simulink model "mavsim"  (R2020a)
settings: Solver=ode45  StartTime=0.0  StopTime=500  RelTol=1e-3  EnableMultiTasking=on
PreLoadFcn:
  | kalman_covariances
InitFcn:
  | param_quad
model workspace (MAT data in the model file):
  traj_x = [0 0.201 0.4 0.601 0.8 1 1.2 1.4 1.6 1.801 2 2.2 ... (4684 elements, 2342x2)]
  traj_y = [0 0.201 0.4 0.601 0.8 1 1.2 1.4 1.6 1.801 2 2.2 ... (4684 elements, 2342x2)]
  traj_z = [0 0.201 0.4 0.601 0.8 1 1.2 1.4 1.6 1.801 2 2.2 ... (4684 elements, 2342x2)]
  vel_x = [0 0 0.201 0.4 0.601 0.8 1 1.2 1.4 1.6 1.801 2 ... (4686 elements, 2343x2)]
  vel_y = [0 0 0.201 0.4 0.601 0.8 1 1.2 1.4 1.6 1.801 2 ... (4686 elements, 2343x2)]
  vel_z = [0 0 0.201 0.4 0.601 0.8 1 1.2 1.4 1.6 1.801 2 ... (4686 elements, 2343x2)]
undefined symbols (not defined in the file or in its folder): airdata, drawAircraft, P, plotmavstatevariables
libraries: simulink x5, sharedTrackingLibrary x1
(part 2 of 2)

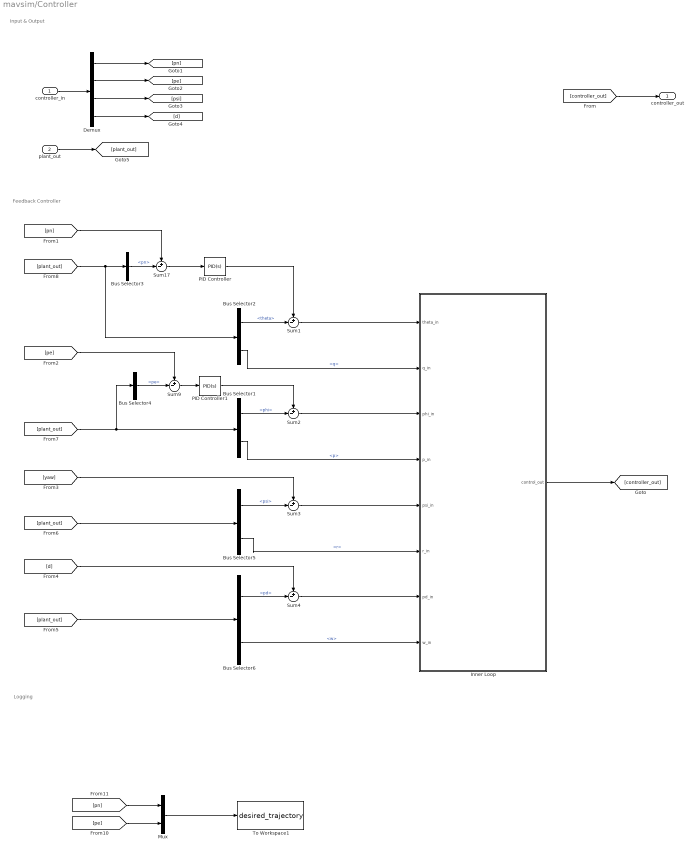
== system mavsim/Controller ==
  note: Logging
  note: Input & Output
  note: Feedback Controller
  controller_in : Inport
  plant_out : Inport  Port=2
  Bus Selector1 : BusSelector  OutputSignals=phi,p
  Bus Selector2 : BusSelector  OutputSignals=theta,q
  Bus Selector3 : BusSelector  OutputSignals=pn
  Bus Selector4 : BusSelector  OutputSignals=pe
  Bus Selector5 : BusSelector  OutputSignals=psi,r
  Bus Selector6 : BusSelector  OutputSignals=pd,w
  Demux : Demux
  Inner Loop : Subsystem
  Mux : Mux  Inputs=2
  PID Controller : simulink/Continuous/PID Controller  Controller=PID  Form=Parallel  TimeDomain=Continuous-time  UseExternalTs=off  SampleTime=1  IntegratorMethod=Forward Euler  FilterMethod=Forward Euler  ControllerParametersSource=internal  P=4.0023736850835e-05  I=2.85008847395968e-08  D=0.0124881440151142  UseFilter=on  N=13.9495577511828  TunerSelectOption=Transfer Function Based (PID Tuner App)  InitialConditionSource=internal  InitialConditionForIntegrator=0  InitialConditionForFilter=0  DifferentiatorICPrevScaledInput=0  ExternalReset=none  TrackingMode=off  Kt=1  LimitOutput=off  UpperSaturationLimit=inf  LowerSaturationLimit=-inf  LinearizeAsGain=on  AntiWindupMode=none  Kb=1  POutMin=[]  POutMax=[]  IOutMin=[]  IOutMax=[]  DOutMin=[]  DOutMax=[]  NOutMin=[]  NOutMax=[]  SumOutMin=[]  SumOutMax=[]  SaturationOutMin=[]  SaturationOutMax=[]  PParamMin=[]  PParamMax=[]  IParamMin=[]  IParamMax=[]  DParamMin=[]  DParamMax=[]  NParamMin=[]  NParamMax=[]  KbParamMin=[]  KbParamMax=[]  KtParamMin=[]  KtParamMax=[]  KbOutMin=[]  KbOutMax=[]  KtOutMin=[]  KtOutMax=[]  IntegratorOutMin=[]  IntegratorOutMax=[]  FilterOutMin=[]  FilterOutMax=[]  SumI1OutMin=[]  SumI1OutMax=[]  SumI2OutMin=[]  SumI2OutMax=[]  SumI3OutMin=[]  SumI3OutMax=[]  SumI4OutMin=[]  SumI4OutMax=[]  SumDOutMin=[]  SumDOutMax=[]  DifferentiatorOutMin=[]  DifferentiatorOutMax=[]  FilterDiffOutCoefMin=[]  FilterDiffOutCoefMax=[]  ReciprocalOutMin=[]  ReciprocalOutMax=[]  SumDenOutMin=[]  SumDenOutMax=[]  SumNumOutMin=[]  SumNumOutMax=[]  DivideOutMin=[]  DivideOutMax=[]  UdiffTsProdOutMin=[]  UdiffTsProdOutMax=[]  NTsProdOutMin=[]  NTsProdOutMax=[]  UintegralTsProdOutMin=[]  UintegralTsProdOutMax=[]  UngainTsProdOutMin=[]  UngainTsProdOutMax=[]  IntegratorContinuousStateAttributes=''  IntegratorStateMustResolveToSignalObject=off  IntegratorRTWStateStorageClass=Auto  FilterContinuousStateAttributes=''  FilterStateMustResolveToSignalObject=off  FilterRTWStateStorageClass=Auto  ParallelPVariant=InternalParameters  IdealPVariant=Disabled  IVariant=InternalParameters  DVariant=InternalParameters  IntegratorVariant=Continuous  SatVariant=Disabled  AWVariant=Passthrough  PCopyVariant=Disabled  TRVariant=Disabled  FdbkBlocksVariant=Forward  IdealPFdbkVariant=Disabled  SatFdbkVariant=Disabled  DerivativeFilterVariant=ContFilter  NVariant=InternalParameters  NCopyVariant=Disabled  FilterICVariant=InternalICsFilter  IntegratorICVariant=InternalICs  ExternalResetVariant=Disabled  TRSumVariant=Passthrough  SumFdbkVariant=Disabled  SumVariant=Sum_PID  TsampFilterVariant=InternalTs  TsampNgainVariant=Passthrough  TsampIntegralVariant=Passthrough
  PID Controller1 : simulink/Continuous/PID Controller  Controller=PID  Form=Parallel  TimeDomain=Continuous-time  UseExternalTs=off  SampleTime=1  IntegratorMethod=Forward Euler  FilterMethod=Forward Euler  ControllerParametersSource=internal  P=-3.61891016622515e-05  I=-2.46103907876315e-08  D=-0.0118238269942865  UseFilter=on  N=13.3217242306574  TunerSelectOption=Transfer Function Based (PID Tuner App)  InitialConditionSource=internal  InitialConditionForIntegrator=0  InitialConditionForFilter=0  DifferentiatorICPrevScaledInput=0  ExternalReset=none  TrackingMode=off  Kt=1  LimitOutput=off  UpperSaturationLimit=inf  LowerSaturationLimit=-inf  LinearizeAsGain=on  AntiWindupMode=none  Kb=1  POutMin=[]  POutMax=[]  IOutMin=[]  IOutMax=[]  DOutMin=[]  DOutMax=[]  NOutMin=[]  NOutMax=[]  SumOutMin=[]  SumOutMax=[]  SaturationOutMin=[]  SaturationOutMax=[]  PParamMin=[]  PParamMax=[]  IParamMin=[]  IParamMax=[]  DParamMin=[]  DParamMax=[]  NParamMin=[]  NParamMax=[]  KbParamMin=[]  KbParamMax=[]  KtParamMin=[]  KtParamMax=[]  KbOutMin=[]  KbOutMax=[]  KtOutMin=[]  KtOutMax=[]  IntegratorOutMin=[]  IntegratorOutMax=[]  FilterOutMin=[]  FilterOutMax=[]  SumI1OutMin=[]  SumI1OutMax=[]  SumI2OutMin=[]  SumI2OutMax=[]  SumI3OutMin=[]  SumI3OutMax=[]  SumI4OutMin=[]  SumI4OutMax=[]  SumDOutMin=[]  SumDOutMax=[]  DifferentiatorOutMin=[]  DifferentiatorOutMax=[]  FilterDiffOutCoefMin=[]  FilterDiffOutCoefMax=[]  ReciprocalOutMin=[]  ReciprocalOutMax=[]  SumDenOutMin=[]  SumDenOutMax=[]  SumNumOutMin=[]  SumNumOutMax=[]  DivideOutMin=[]  DivideOutMax=[]  UdiffTsProdOutMin=[]  UdiffTsProdOutMax=[]  NTsProdOutMin=[]  NTsProdOutMax=[]  UintegralTsProdOutMin=[]  UintegralTsProdOutMax=[]  UngainTsProdOutMin=[]  UngainTsProdOutMax=[]  IntegratorContinuousStateAttributes=''  IntegratorStateMustResolveToSignalObject=off  IntegratorRTWStateStorageClass=Auto  FilterContinuousStateAttributes=''  FilterStateMustResolveToSignalObject=off  FilterRTWStateStorageClass=Auto  ParallelPVariant=InternalParameters  IdealPVariant=Disabled  IVariant=InternalParameters  DVariant=InternalParameters  IntegratorVariant=Continuous  SatVariant=Disabled  AWVariant=Passthrough  PCopyVariant=Disabled  TRVariant=Disabled  FdbkBlocksVariant=Forward  IdealPFdbkVariant=Disabled  SatFdbkVariant=Disabled  DerivativeFilterVariant=ContFilter  NVariant=InternalParameters  NCopyVariant=Disabled  FilterICVariant=InternalICsFilter  IntegratorICVariant=InternalICs  ExternalResetVariant=Disabled  TRSumVariant=Passthrough  SumFdbkVariant=Disabled  SumVariant=Sum_PID  TsampFilterVariant=InternalTs  TsampNgainVariant=Passthrough  TsampIntegralVariant=Passthrough
  Sum{1..4,9,17} (6 alike) : Sum  Inputs=+-|
  To Workspace1 : ToWorkspace  VariableName=desired_trajectory  SaveFormat=Timeseries  SampleTime=-1
  controller_out : Outport  VectorParamsAs1DForOutWhenUnconnected=off
  wires:
  [yaw] -> Sum3/1
  [d] -> Sum4/1
  Bus Selector2/1 -> Sum1/2  "<theta>"
  Bus Selector4/1 -> Sum9/2  "<pe>"
  Sum2/1 -> Inner Loop/3(phi_in)
  Sum4/1 -> Inner Loop/7(pd_in)
  PID Controller/1 -> Sum1/1
  Bus Selector2/2 -> Inner Loop/2(q_in)  "<q>"
  Sum17/1 -> PID Controller/1
  Bus Selector5/1 -> Sum3/2  "<psi>"
  Bus Selector6/2 -> Inner Loop/8(w_in)  "<w>"
  Inner Loop/1(control_out) -> [controller_out]
  Bus Selector1/2 -> Inner Loop/4(p_in)  "<p>"
  [pn] -> Sum17/1
  PID Controller1/1 -> Sum2/1
  Sum9/1 -> PID Controller1/1
  Bus Selector1/1 -> Sum2/2  "<phi>"
  Sum1/1 -> Inner Loop/1(theta_in)
  [plant_out] -> Bus Selector6/1
  [pe] -> Sum9/1
  Sum3/1 -> Inner Loop/5(psi_in)
  Bus Selector6/1 -> Sum4/2  "<pd>"
  Bus Selector5/2 -> Inner Loop/6(r_in)  "<r>"
  Bus Selector3/1 -> Sum17/2  "<pn>"
  [controller_out] -> controller_out/1
  Demux/1 -> [pn]
  Demux/2 -> [pe]
  Demux/3 -> [psi]
  Demux/4 -> [d]
  plant_out/1 -> [plant_out]
  [plant_out] -> Bus Selector5/1
  [plant_out] -> Bus Selector4/1, Bus Selector1/1
  [plant_out] -> Bus Selector2/1, Bus Selector3/1
  controller_in/1 -> Demux/1
  [pe] -> Mux/2
  [pn] -> Mux/1
  Mux/1 -> To Workspace1/1

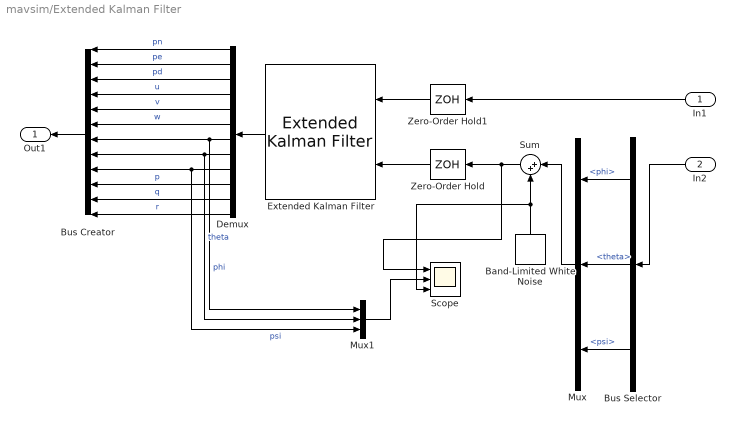
== system mavsim/Extended Kalman Filter ==
  In1 : Inport
  In2 : Inport  Port=2
  Band-Limited White Noise : simulink/Sources/Band-Limited White Noise  Cov=[0.000001 0.000001 0.000001]  Ts=0.005  seed=[23341]
  Bus Creator : BusCreator  Inputs=12
  Bus Selector : BusSelector  OutputSignals=phi,theta,psi
  Demux : Demux  Outputs=12
  Extended Kalman Filter : sharedTrackingLibrary/Extended Kalman Filter  StateTransitionFcn=mavStateTransitionFcn  HasStateTransitionJacobianFcn=off  HasAdditiveProcessNoise=Additive  ProcessNoise=Q  HasTimeVaryingProcessNoise=off  HasStateTransitionFcnExtraArgument=1  InitialState=[0 0 0 0 0 0 0 0 0 0 0 0]  InitialStateCovariance=1e-6  MeasurementFcn1=gyroFcn  HasMeasurementJacobianFcn1=off  HasMeasurementEnablePort1=off  HasAdditiveMeasurementNoise1=Additive  MeasurementNoise1=R  HasTimeVaryingMeasurementNoise1=off  HasMeasurementFcnExtraArgument1=0  MeasurementFcn2=myMeasurementFcn  HasMeasurementJacobianFcn2=off  HasMeasurementEnablePort2=off  HasAdditiveMeasurementNoise2=Additive  MeasurementNoise2=1  HasTimeVaryingMeasurementNoise2=off  HasMeasurementFcnExtraArgument2=0  MeasurementFcn3=myMeasurementFcn  HasMeasurementJacobianFcn3=off  HasMeasurementEnablePort3=off  HasAdditiveMeasurementNoise3=Additive  MeasurementNoise3=1  HasTimeVaryingMeasurementNoise3=off  HasMeasurementFcnExtraArgument3=0  MeasurementFcn4=myMeasurementFcn  HasMeasurementJacobianFcn4=off  HasMeasurementEnablePort4=off  HasAdditiveMeasurementNoise4=Additive  MeasurementNoise4=1  HasTimeVaryingMeasurementNoise4=off  HasMeasurementFcnExtraArgument4=0  MeasurementFcn5=myMeasurementFcn  HasMeasurementJacobianFcn5=off  HasMeasurementEnablePort5=off  HasAdditiveMeasurementNoise5=Additive  MeasurementNoise5=1  HasTimeVaryingMeasurementNoise5=off  HasMeasurementFcnExtraArgument5=0  EnableMultirate=off  StateTransitionFcnSampleTime=1  MeasurementFcn1SampleTime=1  MeasurementFcn2SampleTime=1  MeasurementFcn3SampleTime=1  MeasurementFcn4SampleTime=1  MeasurementFcn5SampleTime=1  UseCurrentEstimator=on  OutputStateCovariance=off  DataType=double  SampleTime=.005  NumberOfMeasurements=1
      settings: SourceProductBaseCode=CT,DR,TF,ID,NV,AR,RO,VE
  Mux : Mux  Inputs=3
  Mux1 : Mux  Inputs=3
  Scope : Scope  NumInputPorts=3
  Sum : Sum  Inputs=|++
  Zero-Order Hold : ZeroOrderHold  SampleTime=.005
  Zero-Order Hold1 : ZeroOrderHold  SampleTime=.005
  Out1 : Outport  VectorParamsAs1DForOutWhenUnconnected=off
  wires:
  Sum/1 -> Scope/1, Zero-Order Hold/1
  Zero-Order Hold/1 -> Extended Kalman Filter/2
  In2/1 -> Bus Selector/1
  Mux/1 -> Sum/1
  In1/1 -> Zero-Order Hold1/1
  Zero-Order Hold1/1 -> Extended Kalman Filter/1
  Extended Kalman Filter/1 -> Demux/1
  Bus Creator/1 -> Out1/1
  Demux/1 -> Bus Creator/1  "pn"
  Demux/2 -> Bus Creator/2  "pe"
  Demux/3 -> Bus Creator/3  "pd"
  Demux/4 -> Bus Creator/4  "u"
  Demux/5 -> Bus Creator/5  "v"
  Demux/6 -> Bus Creator/6  "w"
  Demux/8 -> Mux1/2, Bus Creator/8  "theta"
  Demux/7 -> Mux1/1, Bus Creator/7  "phi"
  Demux/9 -> Mux1/3, Bus Creator/9  "psi"
  Demux/10 -> Bus Creator/10  "p"
  Demux/11 -> Bus Creator/11  "q"
  Demux/12 -> Bus Creator/12  "r"
  Bus Selector/3 -> Mux/3  "<psi>"
  Bus Selector/1 -> Mux/1  "<phi>"
  Bus Selector/2 -> Mux/2  "<theta>"
  Mux1/1 -> Scope/2
  Band-Limited White Noise/1 -> Scope/3, Sum/2

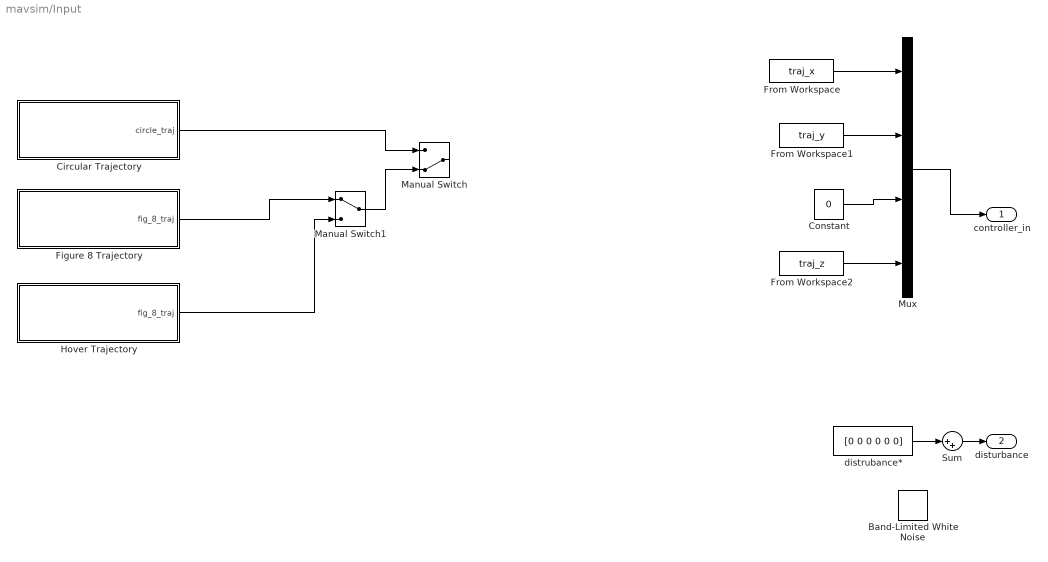
== system mavsim/Input ==
  Band-Limited White Noise : simulink/Sources/Band-Limited White Noise  Cov=[0 0 0 0.0000001 0.0000001 0.0000001]  Ts=0.1  seed=[23341]
  Circular Trajectory : Subsystem
  Constant : Constant  Value=0
  Figure 8 Trajectory : Subsystem
  From Workspace : FromWorkspace  VariableName=traj_x  SampleTime=-1  OutputAfterFinalValue=Holding final value
  From Workspace1 : FromWorkspace  VariableName=traj_y  SampleTime=-1  OutputAfterFinalValue=Holding final value
  From Workspace2 : FromWorkspace  VariableName=traj_z  SampleTime=-1  OutputAfterFinalValue=Holding final value
  Hover Trajectory : Subsystem
  Manual Switch : ManualSwitch  CurrentSetting=0
  Manual Switch1 : ManualSwitch
  Mux : Mux
  Sum : Sum  Inputs=|++
  distrubance* : Constant  Value=[0 0 0 0 0 0]  SampleTime=0
  controller_in : Outport  VectorParamsAs1DForOutWhenUnconnected=off
  disturbance : Outport  Port=2  VectorParamsAs1DForOutWhenUnconnected=off
  wires:
  Circular Trajectory/1(circle_traj) -> Manual Switch/1
  Mux/1 -> controller_in/1
  Sum/1 -> disturbance/1
  distrubance*/1 -> Sum/1
  Figure 8 Trajectory/1(fig_8_traj) -> Manual Switch1/1
  Hover Trajectory/1(fig_8_traj) -> Manual Switch1/2
  Manual Switch1/1 -> Manual Switch/2
  From Workspace2/1 -> Mux/4
  Constant/1 -> Mux/3
  From Workspace1/1 -> Mux/2
  From Workspace/1 -> Mux/1

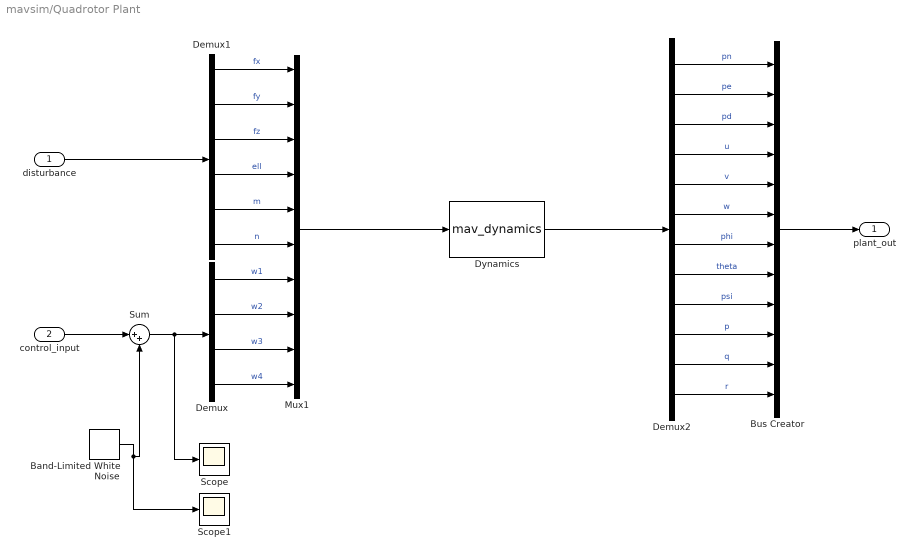
== system mavsim/Quadrotor Plant ==
  disturbance : Inport
  control_input : Inport  Port=2
  Band-Limited White Noise : simulink/Sources/Band-Limited White Noise  Cov=[0.000000009]  Ts=0.005  seed=[23341 4 973 66668]
  Bus Creator : BusCreator  Inputs=12
  Demux : Demux
  Demux1 : Demux  Outputs=6
  Demux2 : Demux  Outputs=12
  Dynamics : S-Function  FunctionName=mav_dynamics  Parameters=P  SFunctionDeploymentMode=off  EnableBusSupport=off
  Mux1 : Mux  Inputs=10
  Scope : Scope
  Scope1 : Scope
  Sum : Sum  Inputs=|++
  plant_out : Outport  VectorParamsAs1DForOutWhenUnconnected=off
  wires:
  Dynamics/1 -> Demux2/1
  Demux2/12 -> Bus Creator/12  "r"
  Demux2/1 -> Bus Creator/1  "pn"
  Demux2/2 -> Bus Creator/2  "pe"
  Demux2/3 -> Bus Creator/3  "pd"
  Demux2/4 -> Bus Creator/4  "u"
  Demux2/5 -> Bus Creator/5  "v"
  Demux2/6 -> Bus Creator/6  "w"
  Demux2/8 -> Bus Creator/8  "theta"
  Demux2/7 -> Bus Creator/7  "phi"
  Demux2/9 -> Bus Creator/9  "psi"
  Demux2/10 -> Bus Creator/10  "p"
  Demux2/11 -> Bus Creator/11  "q"
  Bus Creator/1 -> plant_out/1
  Mux1/1 -> Dynamics/1
  Demux/2 -> Mux1/8  "w2"
  Demux1/5 -> Mux1/5  "m"
  Demux1/4 -> Mux1/4  "ell"
  Demux/4 -> Mux1/10  "w4"
  Demux/1 -> Mux1/7  "w1"
  Demux1/6 -> Mux1/6  "n"
  Demux1/2 -> Mux1/2  "fy"
  Demux1/3 -> Mux1/3  "fz"
  Demux/3 -> Mux1/9  "w3"
  Demux1/1 -> Mux1/1  "fx"
  disturbance/1 -> Demux1/1
  Band-Limited White Noise/1 -> Sum/2, Scope1/1
  control_input/1 -> Sum/1
  Sum/1 -> Scope/1, Demux/1

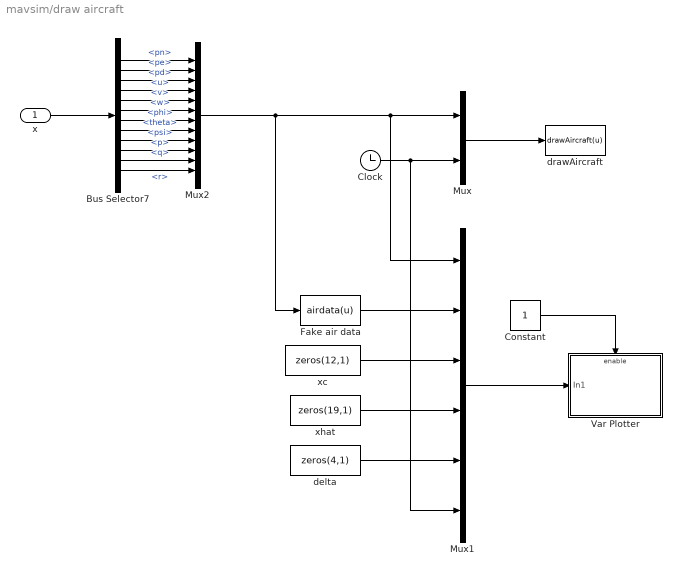
== system mavsim/draw aircraft ==
  x : Inport
  Bus Selector7 : BusSelector  OutputSignals=pn,pe,pd,u,v,w,phi,theta,psi,p,q,r
  Clock : Clock
  Constant : Constant
  Fake air data : MATLABFcn  MATLABFcn=airdata(u)  OutputDimensions=6  SampleTime=0.1
  Mux : Mux  Inputs=2
  Mux1 : Mux  Inputs=6
  Mux2 : Mux  Inputs=12
  Var Plotter : Subsystem
  delta : Constant  Value=zeros(4,1)
  drawAircraft : MATLABFcn  MATLABFcn=drawAircraft(u)  OutputDimensions=0  SampleTime=0.1
  xc : Constant  Value=zeros(12,1)
  xhat : Constant  Value=zeros(19,1)
  wires:
  Mux/1 -> drawAircraft/1
  Mux2/1 -> Fake air data/1, Mux1/1, Mux/1
  Clock/1 -> Mux/2, Mux1/6
  xhat/1 -> Mux1/4
  xc/1 -> Mux1/3
  delta/1 -> Mux1/5
  Fake air data/1 -> Mux1/2
  Mux1/1 -> Var Plotter/1(In1)
  Constant/1 -> Var Plotter/Enable
  Bus Selector7/12 -> Mux2/12  "<r>"
  Bus Selector7/4 -> Mux2/4  "<u>"
  Bus Selector7/9 -> Mux2/9  "<psi>"
  Bus Selector7/5 -> Mux2/5  "<v>"
  Bus Selector7/10 -> Mux2/10  "<p>"
  Bus Selector7/7 -> Mux2/7  "<phi>"
  Bus Selector7/3 -> Mux2/3  "<pd>"
  Bus Selector7/8 -> Mux2/8  "<theta>"
  Bus Selector7/2 -> Mux2/2  "<pe>"
  Bus Selector7/11 -> Mux2/11  "<q>"
  x/1 -> Bus Selector7/1
  Bus Selector7/1 -> Mux2/1  "<pn>"
  Bus Selector7/6 -> Mux2/6  "<w>"

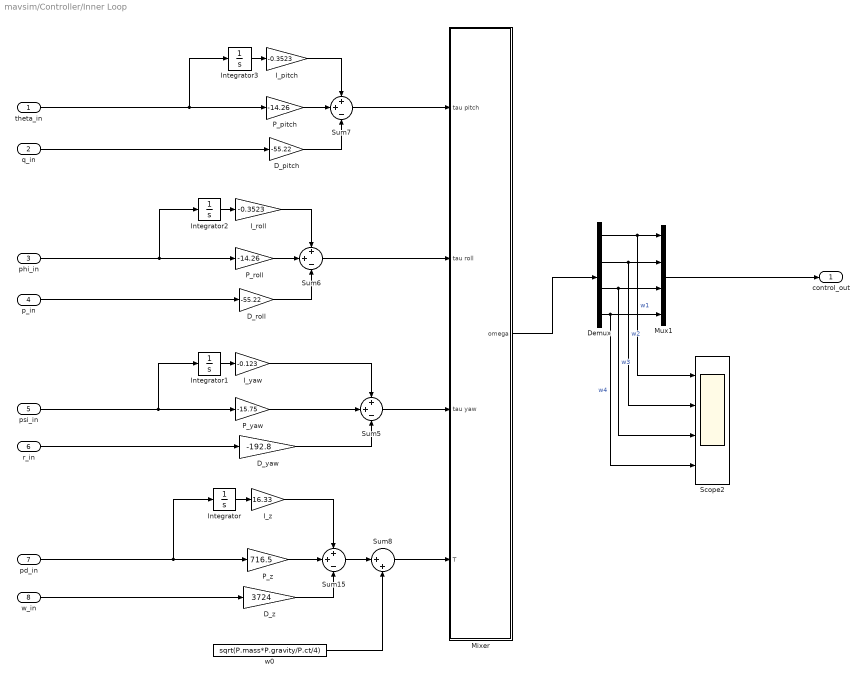
== system mavsim/Controller/Inner Loop ==
  theta_in : Inport
  q_in : Inport  Port=2
  phi_in : Inport  Port=3
  p_in : Inport  Port=4
  psi_in : Inport  Port=5
  r_in : Inport  Port=6
  pd_in : Inport  Port=7
  w_in : Inport  Port=8
  D_pitch : Gain  Gain=-55.22
  D_roll : Gain  Gain=-55.22
  D_yaw : Gain  Gain=-192.8
  D_z : Gain  Gain=3724
  Demux : Demux
  I_pitch : Gain  Gain=-0.3523
  I_roll : Gain  Gain=-0.3523
  I_yaw : Gain  Gain=-0.123
  I_z : Gain  Gain=16.33
  Integrator{,1..3} (4 alike) : Integrator
  Mixer : Subsystem
  Mux1 : Mux
  P_pitch : Gain  Gain=-14.26
  P_roll : Gain  Gain=-14.26
  P_yaw : Gain  Gain=-15.75
  P_z : Gain  Gain=716.5
  Scope2 : Scope  NumInputPorts=4
  Sum{5..7,15} (4 alike) : Sum  Inputs=++-
  Sum8 : Sum  Inputs=|++
  w0 : Constant  Value=sqrt(P.mass*P.gravity/P.ct/4)  SampleTime=0
  control_out : Outport  VectorParamsAs1DForOutWhenUnconnected=off
  wires:
  r_in/1 -> D_yaw/1
  P_pitch/1 -> Sum7/2
  D_yaw/1 -> Sum5/3
  P_roll/1 -> Sum6/2
  Demux/4 -> Mux1/4, Scope2/4  "w4"
  Demux/1 -> Mux1/1, Scope2/1  "w1"
  I_yaw/1 -> Sum5/1
  pd_in/1 -> Integrator/1, P_z/1
  theta_in/1 -> Integrator3/1, P_pitch/1
  Demux/2 -> Mux1/2, Scope2/2  "w2"
  Sum15/1 -> Sum8/1
  I_z/1 -> Sum15/1
  psi_in/1 -> Integrator1/1, P_yaw/1
  Sum8/1 -> Mixer/4(T)
  Mixer/1(omega) -> Demux/1
  phi_in/1 -> Integrator2/1, P_roll/1
  D_roll/1 -> Sum6/3
  Sum7/1 -> Mixer/1(tau pitch)
  Sum5/1 -> Mixer/3(tau yaw)
  Integrator2/1 -> I_roll/1
  Integrator/1 -> I_z/1
  P_yaw/1 -> Sum5/2
  p_in/1 -> D_roll/1
  P_z/1 -> Sum15/2
  Integrator1/1 -> I_yaw/1
  Integrator3/1 -> I_pitch/1
  D_z/1 -> Sum15/3
  D_pitch/1 -> Sum7/3
  Demux/3 -> Mux1/3, Scope2/3  "w3"
  I_pitch/1 -> Sum7/1
  q_in/1 -> D_pitch/1
  w0/1 -> Sum8/2
  I_roll/1 -> Sum6/1
  Mux1/1 -> control_out/1
  Sum6/1 -> Mixer/2(tau roll)
  w_in/1 -> D_z/1

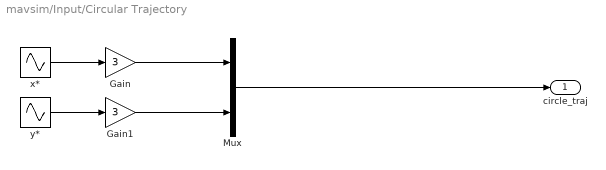
== system mavsim/Input/Circular Trajectory ==
  Gain : Gain  Gain=3
  Gain1 : Gain  Gain=3
  Mux : Mux  Inputs=2
  x* : Sin  Amplitude=50  Frequency=2*pi*.0125  Phase=-pi/2  SampleTime=0
  y* : Sin  Amplitude=50  Frequency=2*pi*.0125  SampleTime=0
  circle_traj : Outport  VectorParamsAs1DForOutWhenUnconnected=off
  wires:
  Mux/1 -> circle_traj/1
  Gain1/1 -> Mux/2
  Gain/1 -> Mux/1
  x*/1 -> Gain/1
  y*/1 -> Gain1/1

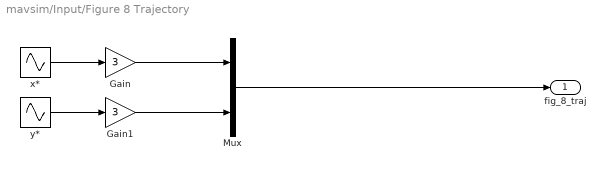
== system mavsim/Input/Figure 8 Trajectory ==
  Gain : Gain  Gain=3
  Gain1 : Gain  Gain=3
  Mux : Mux  Inputs=2
  x* : Sin  Amplitude=50  Frequency=4*pi*.0125  SampleTime=0
  y* : Sin  Amplitude=50  Frequency=2*pi*.0125  SampleTime=0
  fig_8_traj : Outport  VectorParamsAs1DForOutWhenUnconnected=off
  wires:
  Mux/1 -> fig_8_traj/1
  Gain1/1 -> Mux/2
  Gain/1 -> Mux/1
  x*/1 -> Gain/1
  y*/1 -> Gain1/1

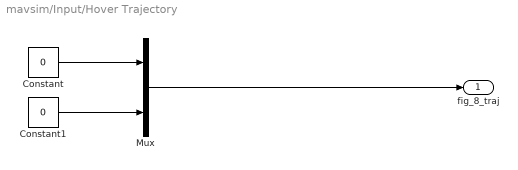
== system mavsim/Input/Hover Trajectory ==
  Constant : Constant  Value=0
  Constant1 : Constant  Value=0
  Mux : Mux  Inputs=2
  fig_8_traj : Outport  VectorParamsAs1DForOutWhenUnconnected=off
  wires:
  Mux/1 -> fig_8_traj/1
  Constant/1 -> Mux/1
  Constant1/1 -> Mux/2

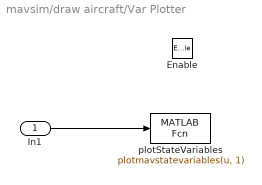
== system mavsim/draw aircraft/Var Plotter ==
  In1 : Inport
  Enable : EnablePort
  plotStateVariables : MATLABFcn  MATLABFcn=plotmavstatevariables(u, 1)  OutputDimensions=0  SampleTime=0.1
  wires:
  In1/1 -> plotStateVariables/1

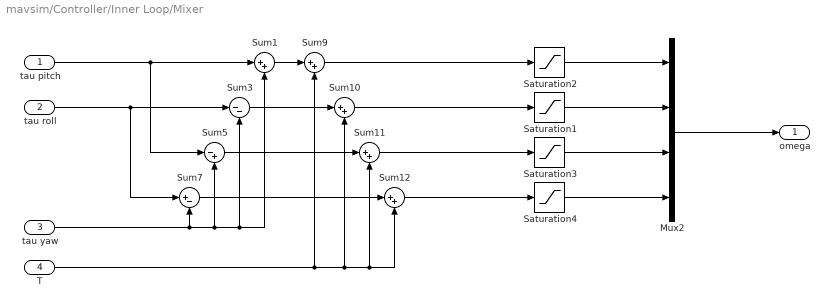
== system mavsim/Controller/Inner Loop/Mixer ==
  tau pitch : Inport
  tau roll : Inport  Port=2
  tau yaw : Inport  Port=3
  T : Inport  Port=4
  Mux2 : Mux
  Saturation{1..4} (4 alike) : Saturate  UpperLimit=8000  LowerLimit=700
  Sum{1,9..12} (5 alike) : Sum  Inputs=|++  InputSameDT=on  SaturateOnIntegerOverflow=on  OutDataTypeStr=Inherit: Same as first input
  Sum3 : Sum  Inputs=|--  InputSameDT=on  SaturateOnIntegerOverflow=on  OutDataTypeStr=Inherit: Same as first input
  Sum5 : Sum  Inputs=|-+  InputSameDT=on  SaturateOnIntegerOverflow=on  OutDataTypeStr=Inherit: Same as first input
  Sum7 : Sum  Inputs=|+-  InputSameDT=on  SaturateOnIntegerOverflow=on  OutDataTypeStr=Inherit: Same as first input
  omega : Outport  VectorParamsAs1DForOutWhenUnconnected=off
  wires:
  Mux2/1 -> omega/1
  tau yaw/1 -> Sum7/2, Sum5/2, Sum3/2, Sum1/2
  Saturation2/1 -> Mux2/1
  Saturation1/1 -> Mux2/2
  Saturation3/1 -> Mux2/3
  Saturation4/1 -> Mux2/4
  tau pitch/1 -> Sum1/1, Sum5/1
  Sum1/1 -> Sum9/1
  Sum3/1 -> Sum10/1
  Sum5/1 -> Sum11/1
  Sum7/1 -> Sum12/1
  Sum9/1 -> Saturation2/1
  Sum10/1 -> Saturation1/1
  Sum11/1 -> Saturation3/1
  Sum12/1 -> Saturation4/1
  T/1 -> Sum11/2, Sum12/2, Sum10/2, Sum9/2
  tau roll/1 -> Sum3/1, Sum7/1
